simulink model "nmpc_block"  (R2019b)
settings: Solver=ode45  StartTime=0.0  StopTime=tfin  FixedStep=1  RelTol=1e-3  EnableMultiTasking=on
values from neighbouring files (symbols this model uses):
  K = nmpc_design(par)    [main_HCW.m]    (also in nmpc_design_template.m)
  ref = [20, 0, 0, 0, 0, 0]    [main_HCW.m]
undefined symbols (not defined in the file or in its folder): constraint_function_template, nmpc_law
libraries: cstblocks x1
settings Model: Creator=carlonovara  LastModifiedBy=user
settings DataIOCC: ReturnWorkspaceOutputs=off
settings OptimizationCC: LifeSpan=inf
settings DebuggingCC: SFUnexpectedBacktrackingDiag=warning  SFNoUnconditionalDefaultTransitionDiag=warning  SFExecutionAtInitializationDiag=none  ArithmeticOperatorsInVariantConditions=warning
settings HardwareCC: ProdBitPerSizeT=32  ProdBitPerPtrDiffT=32  ProdWordSize=32  ProdHWDeviceType=Specified
settings SFSimCC: SimUseLocalCustomCode=off  CustomCodeUndefinedFunction=UseInterfaceOnly
settings RTWCC: RTWUseLocalCustomCode=off
settings CodeAppCC: StateflowObjectComments=on
settings GRTTargetCC: TargetLangStandard=C89/C90 (ANSI)  GeneratePreprocessorConditionals=Disable all
settings ConfigComp: CovMetricSettings=dw  CovHtmlReporting=on  CovSaveCumulativeToWorkspaceVar=on  CovSaveSingleToWorkspaceVar=on  CovExternalEMLEnable=off

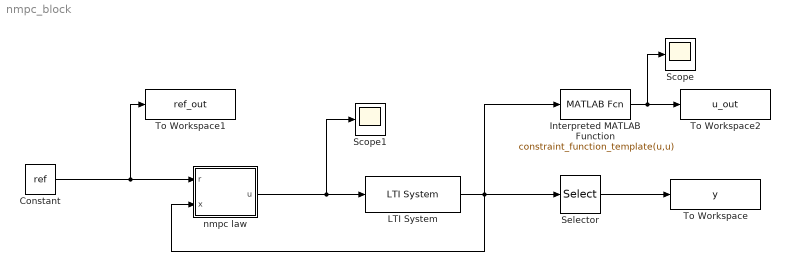
== system nmpc_block ==
  Constant : Constant  Value=ref
  Interpreted MATLAB Function : MATLABFcn  MATLABFcn=constraint_function_template(u,u)
  LTI System : cstblocks/LTI System  sys=H  IC=x0
  Scope : Scope
  Scope1 : Scope
  Selector : Selector  InputPortWidth=6  IndexOptions=Index vector (dialog)  Indices=1:3  OutputSizes=1
  To Workspace : ToWorkspace  VariableName=y  SaveFormat=Timeseries  SampleTime=-1
  To Workspace1 : ToWorkspace  VariableName=ref_out  SaveFormat=Timeseries  SampleTime=-1
  To Workspace2 : ToWorkspace  VariableName=u_out  SaveFormat=Timeseries  SampleTime=-1
  nmpc law : Subsystem
  wires:
  nmpc law/1(u) -> Scope1/1, LTI System/1
  LTI System/1 -> Interpreted MATLAB Function/1, nmpc law/2(x), Selector/1
  Constant/1 -> To Workspace1/1, nmpc law/1(r)
  Selector/1 -> To Workspace/1
  Interpreted MATLAB Function/1 -> Scope/1, To Workspace2/1

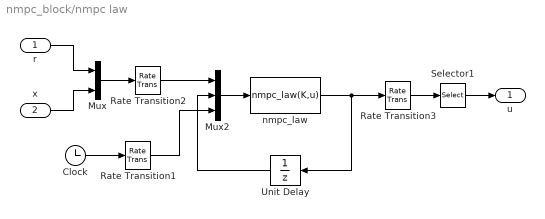
== system nmpc_block/nmpc law ==
  r : Inport
  x : Inport  Port=2
  Clock : Clock
  Mux : Mux  Inputs=2
  Mux2 : Mux  Inputs=3
  Rate Transition1 : RateTransition  OutPortSampleTime=K.Ts
  Rate Transition2 : RateTransition  OutPortSampleTime=K.Ts
  Rate Transition3 : RateTransition  OutPortSampleTime=0
  Selector1 : Selector  InputPortWidth=K.nc  IndexOptions=Index vector (dialog)  Indices=1:K.nu  OutputSizes=1
  Unit Delay : UnitDelay  InitialCondition=zeros(K.nc,1)  SampleTime=K.Ts  HasFrameUpgradeWarning=on
  nmpc_law : MATLABFcn  MATLABFcn=nmpc_law(K,u)  OutputDimensions=K.nc
  u : Outport  VectorParamsAs1DForOutWhenUnconnected=off
  wires:
  Rate Transition3/1 -> Selector1/1
  Unit Delay/1 -> Mux2/2
  Mux2/1 -> nmpc_law/1
  Rate Transition2/1 -> Mux2/1
  nmpc_law/1 -> Rate Transition3/1, Unit Delay/1
  Mux/1 -> Rate Transition2/1
  r/1 -> Mux/1
  x/1 -> Mux/2
  Selector1/1 -> u/1
  Rate Transition1/1 -> Mux2/3
  Clock/1 -> Rate Transition1/1
